simulink model "bolometer"  (R2024a)
settings: Solver=VariableStepAuto  StartTime=0.0  StopTime=10.0  RelTol=1e-3
libraries: spsVoltageMeasurementLib x4, spsParallelRLCBranchLib x2, spsControlledVoltageSourceLib x2, spsControlledCurrentSourceLib x2, spspowerguiLib x1
settings Model: Creator=shubh  LastModifiedBy=shubh

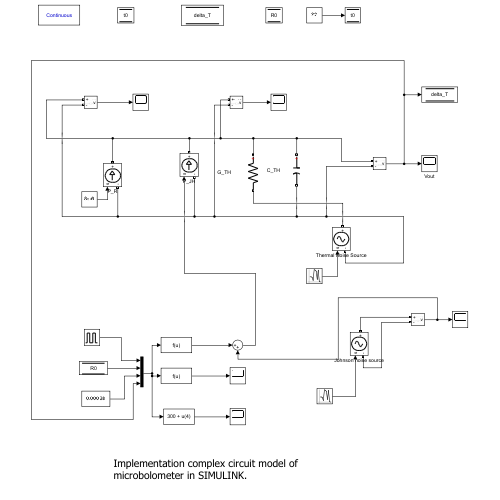
[thumbnail: Simulink's stored preview of the top-level diagram]
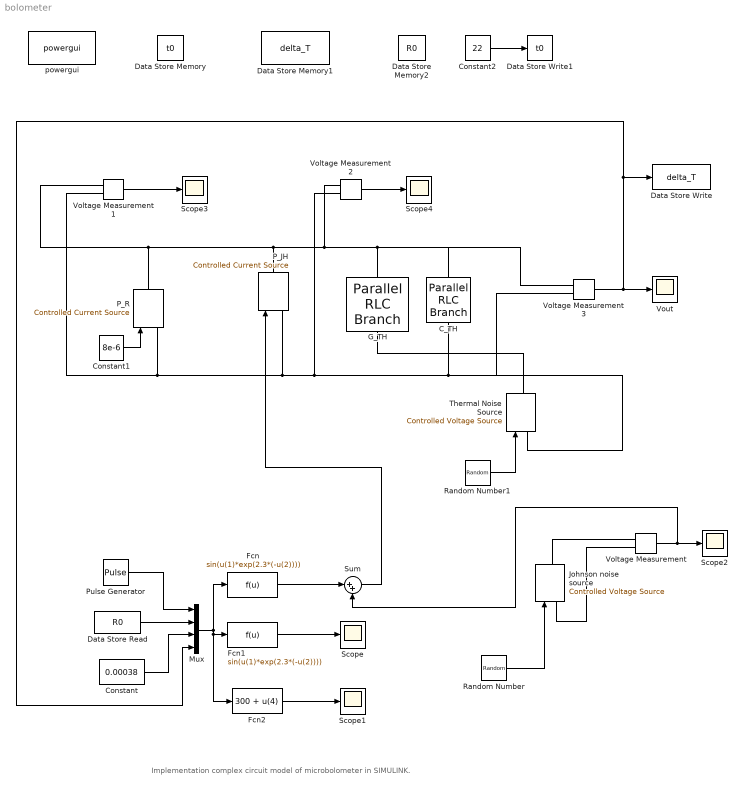
== system bolometer ==
  note: Implementation complex circuit model of microbolometer in SIMULINK.
  C_TH : spsParallelRLCBranchLib/Parallel RLC Branch  LConnTagsString=a  RConnTagsString=__new0  BranchType=C  Resistance=1  Inductance=1e-3  SetiL0=off  InitialCurrent=0  Capacitance=125e-08  Setx0=off  InitialVoltage=0  Measurements=None
  Constant : Constant  Value=0.00038
  Constant1 : Constant  Value=8e-6
  Constant2 : Constant  Value=22
  Data Store Memory : DataStoreMemory  DataStoreName=t0  WriteAfterWriteMsg=warning  ShowAdditionalParam=off
  Data Store Memory1 : DataStoreMemory  DataStoreName=delta_T  WriteAfterWriteMsg=warning  ShowAdditionalParam=off
  Data Store Memory2 : DataStoreMemory  DataStoreName=R0  WriteAfterWriteMsg=warning  ShowAdditionalParam=off
  Data Store Read : DataStoreRead  DataStoreName=R0  IndexOptions=Index vector (dialog)  Indices=1  OutputSizes=1
  Data Store Write : DataStoreWrite  DataStoreName=delta_T  IndexOptions=Index vector (dialog)  Indices=1  OutputSizes=1
  Data Store Write1 : DataStoreWrite  DataStoreName=t0  IndexOptions=Index vector (dialog)  Indices=1  OutputSizes=1
  Fcn : Fcn  Expr=sin(u(1)*exp(2.3*(-u(2))))
  Fcn1 : Fcn  Expr=sin(u(1)*exp(2.3*(-u(2))))
  Fcn2 : Fcn  Expr=300 + u(4)
  G_TH : spsParallelRLCBranchLib/Parallel RLC Branch  LConnTagsString=a  RConnTagsString=__new0  BranchType=R  Resistance=106e-05  Inductance=1e-3  SetiL0=off  InitialCurrent=0  Capacitance=1e-6  Setx0=off  InitialVoltage=0  Measurements=None
  Johnson noise source : spsControlledVoltageSourceLib/Controlled Voltage Source  Initialize=on  Source_Type=AC  Amplitude=7.6e-06  Phase=0  Frequency=0  Measurements=Voltage
  Mux : Mux
  P_JH : spsControlledCurrentSourceLib/Controlled Current Source  Initialize=on  Source_Type=AC  Amplitude=0  Phase=0  Frequency=0  Measurements=None
  P_R : spsControlledCurrentSourceLib/Controlled Current Source  Initialize=on  Source_Type=AC  Amplitude=0  Phase=0  Frequency=0  Measurements=None
  Pulse Generator : DiscretePulseGenerator  PulseType=Time based  Amplitude=0.5  Period=0.1  PulseWidth=50
  Random Number : RandomNumber  Variance=5.8e-11  Seed=123  SampleTime=1e-06
  Random Number1 : RandomNumber  Variance=1e-06  SampleTime=1e-06
  Scope{,1..4} (5 alike) : Scope
  Sum : Sum  Inputs=|++
  Thermal Noise Source : spsControlledVoltageSourceLib/Controlled Voltage Source  Initialize=on  Source_Type=AC  Amplitude=0  Phase=0  Frequency=0  Measurements=None
  Voltage Measurement{,1..3} (4 alike) : spsVoltageMeasurementLib/Voltage Measurement  PhasorSimulation=off  OutputType=Complex  PSBequivalent=0
  Vout : Scope
  powergui : spspowerguiLib/powergui  Priority=1  SimulationMode=Continuous  SampleTime=50e-6  frequency=60  Iterations=50  frequencyindice=0  Pbase=100e6  ErrMax=1e-4  UnitsV=kV  UnitsW=MW  buscounter=0  FunctionMessages=off  echomessages=off  EnableUseOfTLC=off  CurrentSourceSwitches=off  DisableSnubberDevices=off  DisableRonSwitches=off  DisableVfSwitches=off  DisplayEquations=off  AutomaticDiscreteSolvers=off  SolverType=Tustin/Backward Euler (TBE)  Interpol=off  ExternalGateDelay=off  methode=off  Ts=100  x0status=blocks  SPID=on  SwTol=0  HookPort=off  NonlinearTolerance=1e-4  nMaxIteration=100  ContinueOnMaxIteration=off  RestoreLinks=warning  ResistiveCurrentMeasurement=off  Frange=[0:2:500]  Ylog=off  Xlog=on  ShowGrid=off  save=off  variable=ZData  structure=0  ZoomFFT=off  StartTime=0.0  cycles=1  DisplayStyle=1  fundamental=60  FreqAxis=off  MaxFrequency=1000  frequencyindicesteady=1  RmsSteady=1  display=off
  wires:
  Pulse Generator/1 -> Mux/1
  Data Store Read/1 -> Mux/2
  Constant/1 -> Mux/3
  Mux/1 -> Fcn2/1, Fcn1/1, Fcn/1
  Fcn1/1 -> Scope/1
  Fcn2/1 -> Scope1/1
  Fcn/1 -> Sum/1
  Random Number/1 -> Johnson noise source/1
  Random Number1/1 -> Thermal Noise Source/1
  Constant1/1 -> P_R/1
  Voltage Measurement1/1 -> Scope3/1
  Voltage Measurement2/1 -> Scope4/1
  Voltage Measurement3/1 -> Data Store Write/1, Mux/4, Vout/1
  Sum/1 -> P_JH/1
  Voltage Measurement/1 -> Sum/2, Scope2/1
  Constant2/1 -> Data Store Write1/1
  connections:
  Johnson noise source/RConn1 -- Voltage Measurement/LConn1
  Johnson noise source/LConn1 -- Voltage Measurement/LConn2
  P_R/LConn1 -- C_TH/RConn1 -- Voltage Measurement3/LConn2 -- Thermal Noise Source/LConn1 -- Voltage Measurement2/LConn2 -- P_JH/LConn1 -- Voltage Measurement1/LConn2
  P_R/RConn1 -- Voltage Measurement3/LConn1 -- C_TH/LConn1 -- G_TH/LConn1 -- Voltage Measurement2/LConn1 -- P_JH/RConn1 -- Voltage Measurement1/LConn1
  G_TH/RConn1 -- Thermal Noise Source/RConn1
